simulink model "AirHt_Ctl"  (R2016b)
settings: configuration reference "CodeGenConfigSet" (kept outside this file)
values from neighbouring files (symbols this model uses):
  AirHt_bCEngDsT_C = Calibration.Parameter    [init_AirHt_Ctl.m]    (also in init_AirHt_Ctl_SIL.m = Simulink.Parameter)
  AirHt_bEnvT_C = Calibration.Parameter    [init_AirHt_Ctl.m]    (also in init_AirHt_Ctl_SIL.m = Simulink.Parameter)
  AirHt_bFuelT_C = Calibration.Parameter    [init_AirHt_Ctl.m]    (also in init_AirHt_Ctl_SIL.m = Simulink.Parameter)
  AirHt_bOilT_C = Calibration.Parameter    [init_AirHt_Ctl.m]    (also in init_AirHt_Ctl_SIL.m = Simulink.Parameter)
  AirHt_btAFS_C = Calibration.Parameter    [init_AirHt_Ctl.m]    (also in init_AirHt_Ctl_SIL.m = Simulink.Parameter)
  AirHt_btCACDs_C = Calibration.Parameter    [init_AirHt_Ctl.m]    (also in init_AirHt_Ctl_SIL.m = Simulink.Parameter)
  AirHt_btIntkVUs_C = Calibration.Parameter    [init_AirHt_Ctl.m]    (also in init_AirHt_Ctl_SIL.m = Simulink.Parameter)
  AIRHT_MAX_TEMP = fi(150,Temp_deg)    [init_AirHt_Ctl.m]    (also in init_AirHt_Ctl_SIL.m)
  AirHt_nMin_C = Calibration.Parameter    [init_AirHt_Ctl.m]    (also in init_AirHt_Ctl_SIL.m = Simulink.Parameter)
  AirHt_referencetemp_C = Calibration.Parameter    [init_AirHt_Ctl.m]    (also in init_AirHt_Ctl_SIL.m = Simulink.Parameter)
  AirHt_tiBlink_C = Calibration.Parameter    [init_AirHt_Ctl.m]    (also in init_AirHt_Ctl_SIL.m = Simulink.Parameter)
  AirHt_tiCrankHt_MAP = Calibration.Parameter    [init_AirHt_Ctl.m]    (also in init_AirHt_Ctl_SIL.m = Simulink.Parameter)
  AirHt_tiCrankHt_MAPX = Calibration.Parameter    [init_AirHt_Ctl.m]    (also in init_AirHt_Ctl_SIL.m = Simulink.Parameter)
  AirHt_tiCrankHt_MAPY = Calibration.Parameter    [init_AirHt_Ctl.m]    (also in init_AirHt_Ctl_SIL.m = Simulink.Parameter)
  AirHt_tiLowBattThr_C = Calibration.Parameter    [init_AirHt_Ctl.m]    (also in init_AirHt_Ctl_SIL.m = Simulink.Parameter)
  AirHt_tiPostHt_MAP = Calibration.Parameter    [init_AirHt_Ctl.m]    (also in init_AirHt_Ctl_SIL.m = Simulink.Parameter)
  AirHt_tiPostHt_MAPX = Calibration.Parameter    [init_AirHt_Ctl.m]    (also in init_AirHt_Ctl_SIL.m = Simulink.Parameter)
  AirHt_tiPostHt_MAPY = Calibration.Parameter    [init_AirHt_Ctl.m]    (also in init_AirHt_Ctl_SIL.m = Simulink.Parameter)
  AirHt_tiPreHt_MAP = Calibration.Parameter    [init_AirHt_Ctl.m]    (also in init_AirHt_Ctl_SIL.m = Simulink.Parameter)
  AirHt_tiPreHt_MAPX = Calibration.Parameter    [init_AirHt_Ctl.m]    (also in init_AirHt_Ctl_SIL.m = Simulink.Parameter)
  AirHt_tiPreHt_MAPY = Calibration.Parameter    [init_AirHt_Ctl.m]    (also in init_AirHt_Ctl_SIL.m = Simulink.Parameter)
  AirHt_tiStByHt_MAP = Calibration.Parameter    [init_AirHt_Ctl.m]    (also in init_AirHt_Ctl_SIL.m = Simulink.Parameter)
  AirHt_tiStByHt_MAPX = Calibration.Parameter    [init_AirHt_Ctl.m]    (also in init_AirHt_Ctl_SIL.m = Simulink.Parameter)
  AirHt_tiStByHt_MAPY = Calibration.Parameter    [init_AirHt_Ctl.m]    (also in init_AirHt_Ctl_SIL.m = Simulink.Parameter)
  AirHt_tiStDelay_C = Calibration.Parameter    [init_AirHt_Ctl.m]    (also in init_AirHt_Ctl_SIL.m = Simulink.Parameter)
  AirHt_uLowBattThr_C = Calibration.Parameter    [init_AirHt_Ctl.m]    (also in init_AirHt_Ctl_SIL.m = Simulink.Parameter)
undefined symbols (not defined in the file or in its folder): AirHt_Ctl_DT, AirHtState_conv, EngState_conv
libraries: CXLib x2
settings Model: Creator=GaberXu  LastModifiedBy=guanxiaoxing
settings ConfigSetRef: SourceLocation=Base Workspace

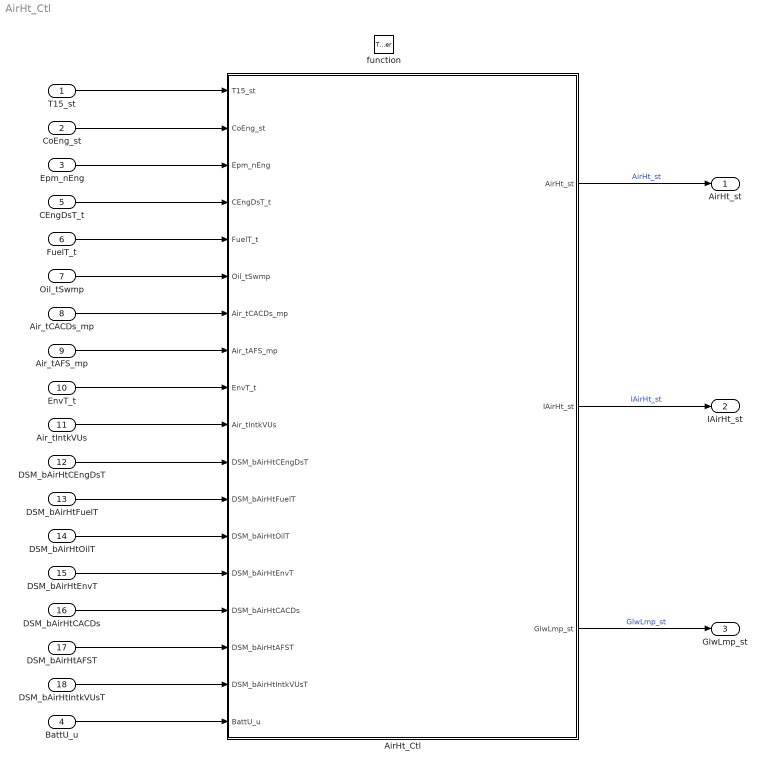
== system AirHt_Ctl ==
  T15_st : Inport  Description=Terminal 15 status after debouncing  OutDataTypeStr=Enum: Switch_conv
  CoEng_st : Inport  Description=Engine coordinator state  Port=2  OutDataTypeStr=Enum: EngState_conv
  Epm_nEng : Inport  Tag=rpm  Description=Engine speed  Port=3  OutMin=0  OutMax=6000  OutDataTypeStr=EngSpeed_rpm
  BattU_u : Inport  Tag=mv  Description=Battery voltage  Port=4  OutMin=0  OutMax=50000  OutDataTypeStr=Battery_mv
  CEngDsT_t : Inport  Tag=deg  Description=engine coolant temperature after filter  Port=5  OutMin=-200  OutMax=200  OutDataTypeStr=Temp_deg
  FuelT_t : Inport  Tag=deg  Description=Temperature of fuel  Port=6  OutMin=-50  OutMax=150  OutDataTypeStr=Temp_deg
  Oil_tSwmp : Inport  Tag=deg  Description=Oil temperature in oil sump  Port=7  OutMin=-50  OutMax=200  OutDataTypeStr=Temp_deg
  Air_tCACDs_mp : Inport  Tag=deg  Description=Charge-air temperature downstream from charge-air cooler  Port=8  OutMin=-200  OutMax=200  OutDataTypeStr=Temp_deg
  Air_tAFS_mp : Inport  Tag=deg  Description=Induction air temperature at the HFM  Port=9  OutMin=-200  OutMax=200  OutDataTypeStr=Temp_deg
  EnvT_t : Inport  Tag=deg  Description=Environmental temperature  Port=10  OutMin=-200  OutMax=200  OutDataTypeStr=Temp_deg
  Air_tIntkVUs : Inport  Tag=deg  Description=Intake air temperature upstream of the inlet valve  Port=11  OutMin=-200  OutMax=200  OutDataTypeStr=Temp_deg
  DSM_bAirHtCEngDsT : Inport  Description=Status of FId_AirHtCEngDsT  Port=12  OutMin=0  OutMax=1  OutDataTypeStr=boolean
  DSM_bAirHtFuelT : Inport  Description=Status of FId_AirHtFuelT  Port=13  OutMin=0  OutMax=1  OutDataTypeStr=boolean
  DSM_bAirHtOilT : Inport  Description=Status of FId_AirHtOilT  Port=14  OutMin=0  OutMax=1  OutDataTypeStr=boolean
  DSM_bAirHtEnvT : Inport  Description=Status of FId_AirHtEnvT_mp  Port=15  OutMin=0  OutMax=1  OutDataTypeStr=boolean
  DSM_bAirHtCACDs : Inport  Description=Status of FId_AirHtCACDs  Port=16  OutMin=0  OutMax=1  OutDataTypeStr=boolean
  DSM_bAirHtAFST : Inport  Description=Status of FId_AirHtAFST  Port=17  OutMin=0  OutMax=1  OutDataTypeStr=boolean
  DSM_bAirHtIntkVUsT : Inport  Description=Status of FId_AirHtntkVUsT  Port=18  OutMin=0  OutMax=1  OutDataTypeStr=boolean
  function : TriggerPort  TriggerType=function-call  VariantControl=Variant  PortDimensions=1
  AirHt_Ctl : Subsystem
  AirHt_st : Outport  Description=status of AirHeater  OutDataTypeStr=Enum: AirHtState_conv
  IAirHt_st : Outport  Description=Request for intake air heater ON/OFF from ASW.  Port=2  OutMin=0  OutMax=1  OutDataTypeStr=boolean
  GlwLmp_st : Outport  Description=Glow lamp status  Port=3  OutMin=0  OutMax=1  OutDataTypeStr=boolean
  wires:
  AirHt_Ctl/1(AirHt_st) -> AirHt_st/1  "AirHt_st"
  AirHt_Ctl/2(IAirHt_st) -> IAirHt_st/1  "IAirHt_st"
  AirHt_Ctl/3(GlwLmp_st) -> GlwLmp_st/1  "GlwLmp_st"
  CoEng_st/1 -> AirHt_Ctl/2(CoEng_st)
  Epm_nEng/1 -> AirHt_Ctl/3(Epm_nEng)
  T15_st/1 -> AirHt_Ctl/1(T15_st)
  BattU_u/1 -> AirHt_Ctl/18(BattU_u)
  CEngDsT_t/1 -> AirHt_Ctl/4(CEngDsT_t)
  DSM_bAirHtIntkVUsT/1 -> AirHt_Ctl/17(DSM_bAirHtIntkVUsT)
  DSM_bAirHtEnvT/1 -> AirHt_Ctl/14(DSM_bAirHtEnvT)
  DSM_bAirHtCACDs/1 -> AirHt_Ctl/15(DSM_bAirHtCACDs)
  Oil_tSwmp/1 -> AirHt_Ctl/6(Oil_tSwmp)
  Air_tAFS_mp/1 -> AirHt_Ctl/8(Air_tAFS_mp)
  DSM_bAirHtAFST/1 -> AirHt_Ctl/16(DSM_bAirHtAFST)
  DSM_bAirHtFuelT/1 -> AirHt_Ctl/12(DSM_bAirHtFuelT)
  FuelT_t/1 -> AirHt_Ctl/5(FuelT_t)
  Air_tIntkVUs/1 -> AirHt_Ctl/10(Air_tIntkVUs)
  Air_tCACDs_mp/1 -> AirHt_Ctl/7(Air_tCACDs_mp)
  EnvT_t/1 -> AirHt_Ctl/9(EnvT_t)
  DSM_bAirHtOilT/1 -> AirHt_Ctl/13(DSM_bAirHtOilT)
  DSM_bAirHtCEngDsT/1 -> AirHt_Ctl/11(DSM_bAirHtCEngDsT)

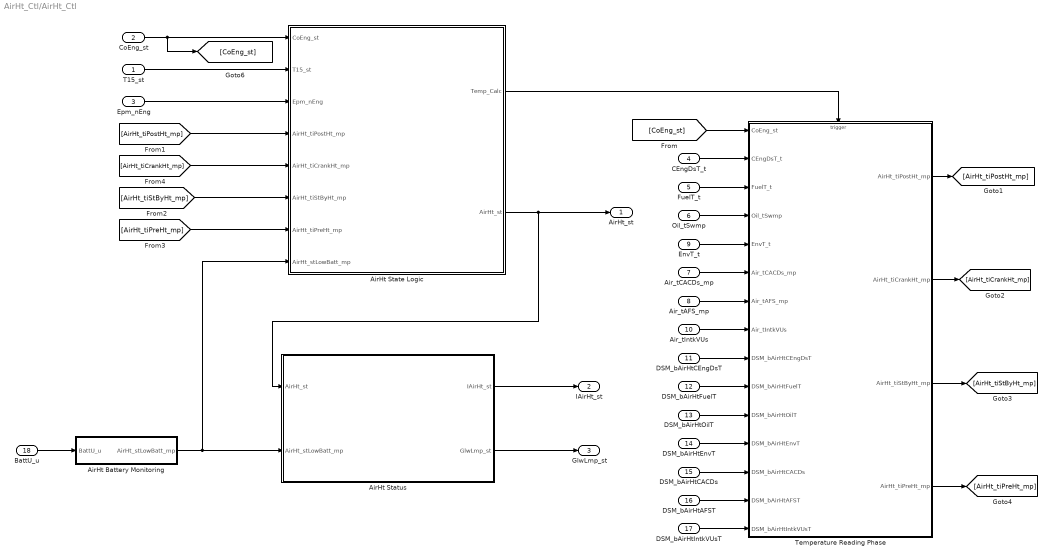
== system AirHt_Ctl/AirHt_Ctl ==
  T15_st : Inport  Description=Terminal 15 status after debouncing
  CoEng_st : Inport  Description=Engine coordinator state  Port=2
  Epm_nEng : Inport  Tag=rpm  Description=Engine speed  Port=3
  CEngDsT_t : Inport  Tag=deg  Description=engine coolant temperature after filter  Port=4  OutMin=-200  OutMax=200  OutDataTypeStr=Temp_deg
  FuelT_t : Inport  Tag=deg  Description=Temperature of fuel  Port=5  OutMin=-50  OutMax=150  OutDataTypeStr=Temp_deg
  Oil_tSwmp : Inport  Tag=deg  Description=Oil temperature in oil sump  Port=6  OutMin=-50  OutMax=200  OutDataTypeStr=Temp_deg
  Air_tCACDs_mp : Inport  Tag=deg  Description=Charge-air temperature downstream from charge-air cooler  Port=7  OutMin=-200  OutMax=200  OutDataTypeStr=Temp_deg
  Air_tAFS_mp : Inport  Tag=deg  Description=Induction air temperature at the HFM  Port=8  OutMin=-200  OutMax=200  OutDataTypeStr=Temp_deg
  EnvT_t : Inport  Tag=deg  Description=Environmental temperature  Port=9  OutMin=-200  OutMax=200  OutDataTypeStr=Temp_deg
  Air_tIntkVUs : Inport  Tag=deg  Description=Intake air temperature upstream of the inlet valve  Port=10  OutMin=-200  OutMax=200  OutDataTypeStr=Temp_deg
  DSM_bAirHtCEngDsT : Inport  Description=Status of FId_AirHtCEngDsT  Port=11  OutMin=0  OutMax=1  OutDataTypeStr=boolean
  DSM_bAirHtFuelT : Inport  Description=Status of FId_AirHtFuelT  Port=12  OutMin=0  OutMax=1  OutDataTypeStr=boolean
  DSM_bAirHtOilT : Inport  Description=Status of FId_AirHtOilT  Port=13  OutMin=0  OutMax=1  OutDataTypeStr=boolean
  DSM_bAirHtEnvT : Inport  Description=Status of FId_AirHtEnvT_mp  Port=14  OutMin=0  OutMax=1  OutDataTypeStr=boolean
  DSM_bAirHtCACDs : Inport  Description=Status of FId_AirHtCACDs  Port=15  OutMin=0  OutMax=1  OutDataTypeStr=boolean
  DSM_bAirHtAFST : Inport  Description=Status of FId_AirHtAFST  Port=16  OutMin=0  OutMax=1  OutDataTypeStr=boolean
  DSM_bAirHtIntkVUsT : Inport  Description=Status of FId_AirHtntkVUsT  Port=17  OutMin=0  OutMax=1  OutDataTypeStr=boolean
  BattU_u : Inport  Tag=mv  Description=Battery voltage  Port=18
  AirHt Battery Monitoring : Subsystem
  AirHt State Logic : Subsystem
  AirHt Status : Subsystem
  Temperature Reading Phase : Subsystem
      settings: RTWFcnNameOpts=User specified  RTWFileNameOpts=User specified
  AirHt_st : Outport  Description=status of AirHeater
  IAirHt_st : Outport  Description=Request for intake air heater ON/OFF from ASW.  Port=2
  GlwLmp_st : Outport  Description=Glow lamp status  Port=3
  wires:
  T15_st/1 -> AirHt State Logic/2(T15_st)
  Epm_nEng/1 -> AirHt State Logic/3(Epm_nEng)
  [AirHt_tiStByHt_mp] -> AirHt State Logic/6(AirHt_tiStByHt_mp)
  [AirHt_tiPostHt_mp] -> AirHt State Logic/4(AirHt_tiPostHt_mp)
  [AirHt_tiCrankHt_mp] -> AirHt State Logic/5(AirHt_tiCrankHt_mp)
  AirHt Status/1(IAirHt_st) -> IAirHt_st/1
  AirHt Status/2(GlwLmp_st) -> GlwLmp_st/1
  CoEng_st/1 -> [CoEng_st], AirHt State Logic/1(CoEng_st)
  Temperature Reading Phase/1(AirHt_tiPostHt_mp) -> [AirHt_tiPostHt_mp]
  Temperature Reading Phase/2(AirHt_tiCrankHt_mp) -> [AirHt_tiCrankHt_mp]
  Temperature Reading Phase/3(AirHt_tiStByHt_mp) -> [AirHt_tiStByHt_mp]
  Temperature Reading Phase/4(AirHt_tiPreHt_mp) -> [AirHt_tiPreHt_mp]
  AirHt State Logic/2(AirHt_st) -> AirHt_st/1, AirHt Status/1(AirHt_st)
  AirHt State Logic/1(Temp_Calc) -> Temperature Reading Phase/Trigger
  [CoEng_st] -> Temperature Reading Phase/1(CoEng_st)
  CEngDsT_t/1 -> Temperature Reading Phase/2(CEngDsT_t)
  DSM_bAirHtOilT/1 -> Temperature Reading Phase/11(DSM_bAirHtOilT)
  DSM_bAirHtCACDs/1 -> Temperature Reading Phase/13(DSM_bAirHtCACDs)
  Oil_tSwmp/1 -> Temperature Reading Phase/4(Oil_tSwmp)
  DSM_bAirHtCEngDsT/1 -> Temperature Reading Phase/9(DSM_bAirHtCEngDsT)
  DSM_bAirHtEnvT/1 -> Temperature Reading Phase/12(DSM_bAirHtEnvT)
  DSM_bAirHtAFST/1 -> Temperature Reading Phase/14(DSM_bAirHtAFST)
  DSM_bAirHtIntkVUsT/1 -> Temperature Reading Phase/15(DSM_bAirHtIntkVUsT)
  DSM_bAirHtFuelT/1 -> Temperature Reading Phase/10(DSM_bAirHtFuelT)
  Air_tIntkVUs/1 -> Temperature Reading Phase/8(Air_tIntkVUs)
  FuelT_t/1 -> Temperature Reading Phase/3(FuelT_t)
  AirHt Battery Monitoring/1(AirHt_stLowBatt_mp) -> AirHt State Logic/8(AirHt_stLowBatt_mp), AirHt Status/2(AirHt_stLowBatt_mp)
  BattU_u/1 -> AirHt Battery Monitoring/1(BattU_u)
  [AirHt_tiPreHt_mp] -> AirHt State Logic/7(AirHt_tiPreHt_mp)
  EnvT_t/1 -> Temperature Reading Phase/5(EnvT_t)
  Air_tAFS_mp/1 -> Temperature Reading Phase/7(Air_tAFS_mp)
  Air_tCACDs_mp/1 -> Temperature Reading Phase/6(Air_tCACDs_mp)

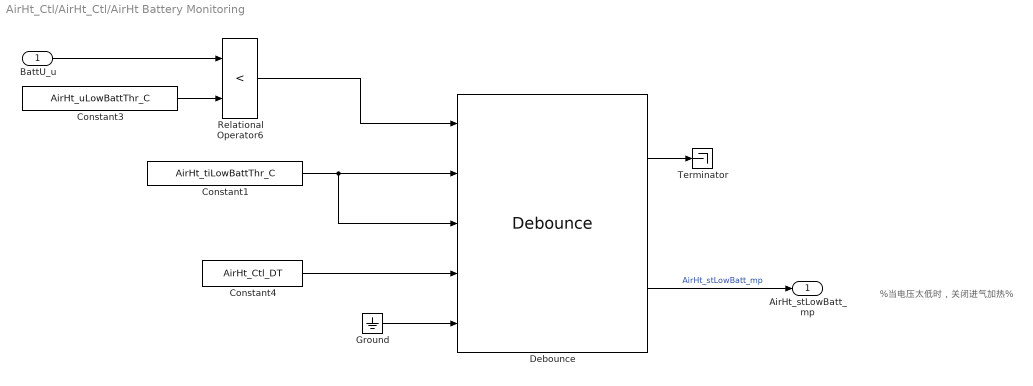
== system AirHt_Ctl/AirHt_Ctl/AirHt Battery Monitoring ==
  note: %当电压太低时，关闭进气加热%
  BattU_u : Inport
  Constant1 : Constant  Value=AirHt_tiLowBattThr_C  SampleTime=-1
  Constant3 : Constant  Value=AirHt_uLowBattThr_C  SampleTime=-1
  Constant4 : Constant  Value=AirHt_Ctl_DT  SampleTime=-1
  Debounce : CXLib/Debounce
  Ground : Ground
  Relational Operator6 : RelationalOperator  Operator=<  OutDataTypeStr=boolean  RndMeth=Simplest  InputSameDT=on
  Terminator : Terminator
  AirHt_stLowBatt_mp : Outport
  wires:
  Relational Operator6/1 -> Debounce/1
  BattU_u/1 -> Relational Operator6/1
  Debounce/1 -> Terminator/1
  Debounce/2 -> AirHt_stLowBatt_mp/1  "AirHt_stLowBatt_mp"
  Constant1/1 -> Debounce/2, Debounce/3
  Ground/1 -> Debounce/5
  Constant3/1 -> Relational Operator6/2
  Constant4/1 -> Debounce/4

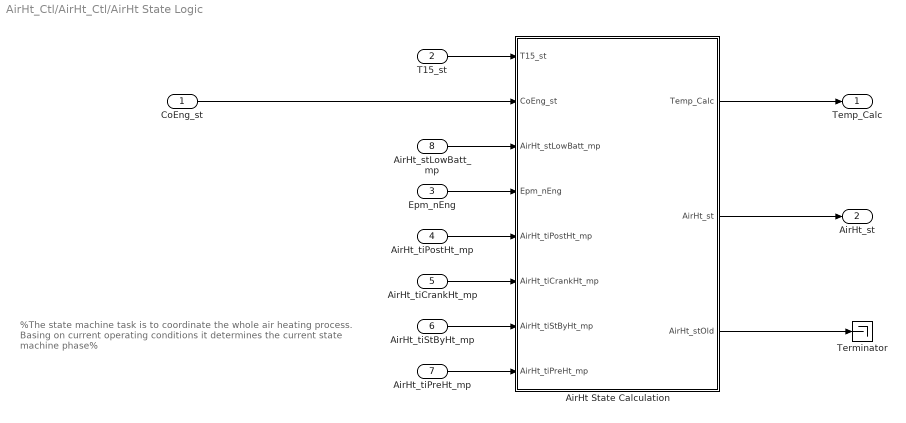
== system AirHt_Ctl/AirHt_Ctl/AirHt State Logic ==
  note: %The state machine task is to coordinate the whole air heating process.
      | Basing on current operating conditions it determines the current state
      | machine phase%
  CoEng_st : Inport
  T15_st : Inport  Port=2
  Epm_nEng : Inport  Port=3
  AirHt_tiPostHt_mp : Inport  Port=4
  AirHt_tiCrankHt_mp : Inport  Port=5
  AirHt_tiStByHt_mp : Inport  Port=6
  AirHt_tiPreHt_mp : Inport  Port=7
  AirHt_stLowBatt_mp : Inport  Port=8
  AirHt State Calculation : Subsystem
      settings: RTWFcnNameOpts=User specified  RTWFileNameOpts=User specified
  Terminator : Terminator
  Temp_Calc : Outport
  AirHt_st : Outport  Port=2
  wires:
  AirHt State Calculation/3(AirHt_stOld) -> Terminator/1
  Epm_nEng/1 -> AirHt State Calculation/4(Epm_nEng)
  AirHt_stLowBatt_mp/1 -> AirHt State Calculation/3(AirHt_stLowBatt_mp)
  T15_st/1 -> AirHt State Calculation/1(T15_st)
  AirHt State Calculation/2(AirHt_st) -> AirHt_st/1
  AirHt_tiPostHt_mp/1 -> AirHt State Calculation/5(AirHt_tiPostHt_mp)
  AirHt_tiCrankHt_mp/1 -> AirHt State Calculation/6(AirHt_tiCrankHt_mp)
  AirHt_tiStByHt_mp/1 -> AirHt State Calculation/7(AirHt_tiStByHt_mp)
  AirHt_tiPreHt_mp/1 -> AirHt State Calculation/8(AirHt_tiPreHt_mp)
  CoEng_st/1 -> AirHt State Calculation/2(CoEng_st)
  AirHt State Calculation/1(Temp_Calc) -> Temp_Calc/1

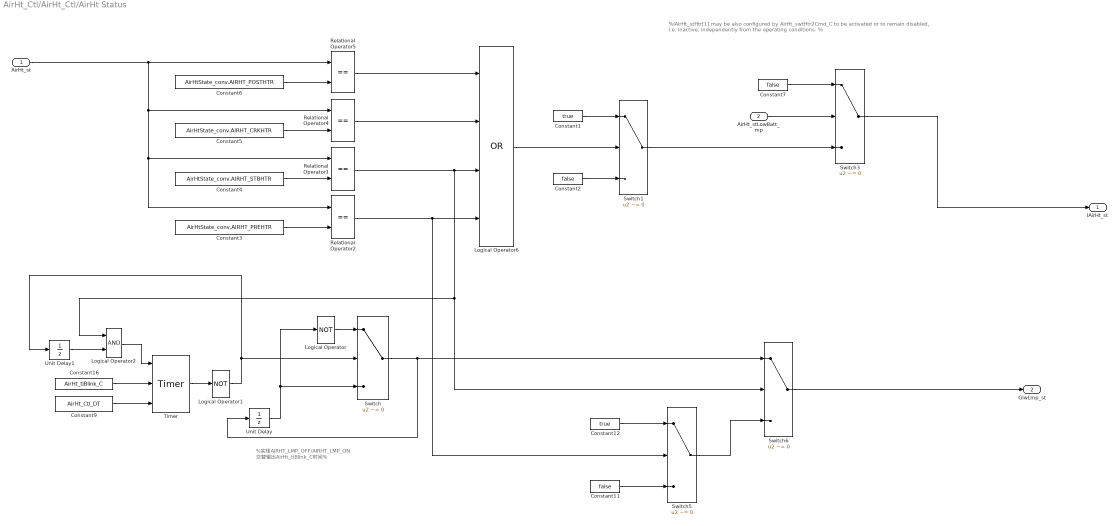
== system AirHt_Ctl/AirHt_Ctl/AirHt Status ==
  note: %实现AIRHT_LMP_OFF/AIRHT_LMP_ON
      | 交替输出AirHt_tiBlink_C时间%
  note: %IAirHt_stHtr[1] may be also configured by AirHt_swtHtr2Cmd_C to be activated or to remain disabled, i.e. inactive, independently
      | from the operating conditions. %
  AirHt_st : Inport
  AirHt_stLowBatt_mp : Inport  Port=2
  Constant1 : Constant  Value=true  OutDataTypeStr=boolean
  Constant11 : Constant  Value=false  OutDataTypeStr=boolean
  Constant12 : Constant  Value=true  OutDataTypeStr=boolean
  Constant16 : Constant  Value=AirHt_tiBlink_C  SampleTime=-1
  Constant2 : Constant  Value=false  OutDataTypeStr=boolean
  Constant3 : Constant  Value=AirHtState_conv.AIRHT_PREHTR  SampleTime=-1
  Constant4 : Constant  Value=AirHtState_conv.AIRHT_STBHTR  SampleTime=-1
  Constant5 : Constant  Value=AirHtState_conv.AIRHT_CRKHTR  SampleTime=-1
  Constant6 : Constant  Value=AirHtState_conv.AIRHT_POSTHTR  SampleTime=-1
  Constant7 : Constant  Value=false  OutDataTypeStr=boolean
  Constant9 : Constant  Value=AirHt_Ctl_DT  SampleTime=-1
  Logical Operator : Logic  Operator=NOT  AllPortsSameDT=off  OutDataTypeStr=boolean
  Logical Operator1 : Logic  Operator=NOT  AllPortsSameDT=off  OutDataTypeStr=boolean
  Logical Operator2 : Logic  AllPortsSameDT=off  OutDataTypeStr=boolean
  Logical Operator6 : Logic  Operator=OR  Inputs=4  OutDataTypeStr=boolean
  Relational Operator{1..2,4..5} (4 alike) : RelationalOperator  Operator===  OutDataTypeStr=boolean  RndMeth=Simplest  InputSameDT=on
  Switch : Switch  Criteria=u2 ~= 0
  Switch1 : Switch  Criteria=u2 ~= 0  InputSameDT=on
  Switch3 : Switch  Criteria=u2 ~= 0  SaturateOnIntegerOverflow=on  InputSameDT=on
  Switch5 : Switch  Criteria=u2 ~= 0  SaturateOnIntegerOverflow=on  InputSameDT=on
  Switch6 : Switch  Criteria=u2 ~= 0  SaturateOnIntegerOverflow=on  InputSameDT=on
  Timer : CXLib/Timer
  Unit Delay : UnitDelay  SampleTime=-1
      settings: AttributesFormatString=InitialValue=%<InitialCondition>
  Unit Delay1 : UnitDelay  SampleTime=-1
      settings: AttributesFormatString=InitialValue=%<InitialCondition>
  IAirHt_st : Outport  Description=Request for intake air heater ON/OFF from ASW.
  GlwLmp_st : Outport  Description=Glow lamp status  Port=2
  wires:
  Switch6/1 -> GlwLmp_st/1
  Switch3/1 -> IAirHt_st/1
  Logical Operator/1 -> Switch/1
  Unit Delay1/1 -> Logical Operator2/2
  Logical Operator1/1 -> Switch/2, Unit Delay1/1
  Switch/1 -> Unit Delay/1, Switch6/1
  Timer/1 -> Logical Operator1/1
  Unit Delay/1 -> Switch/3, Logical Operator/1
  Constant16/1 -> Timer/2
  Constant9/1 -> Timer/3
  AirHt_st/1 -> Relational Operator1/1, Relational Operator2/1, Relational Operator4/1, Relational Operator5/1
  Constant4/1 -> Relational Operator1/2
  Constant3/1 -> Relational Operator2/2
  Constant5/1 -> Relational Operator4/2
  Constant6/1 -> Relational Operator5/2
  Relational Operator5/1 -> Logical Operator6/1
  Logical Operator6/1 -> Switch1/2
  AirHt_stLowBatt_mp/1 -> Switch3/2
  Switch1/1 -> Switch3/3
  Relational Operator2/1 -> Logical Operator6/4, Switch5/2
  Constant11/1 -> Switch5/3
  Constant12/1 -> Switch5/1
  Relational Operator4/1 -> Logical Operator6/2
  Switch5/1 -> Switch6/3
  Constant7/1 -> Switch3/1
  Constant1/1 -> Switch1/1
  Constant2/1 -> Switch1/3
  Relational Operator1/1 -> Logical Operator6/3, Logical Operator2/1, Switch6/2
  Logical Operator2/1 -> Timer/1

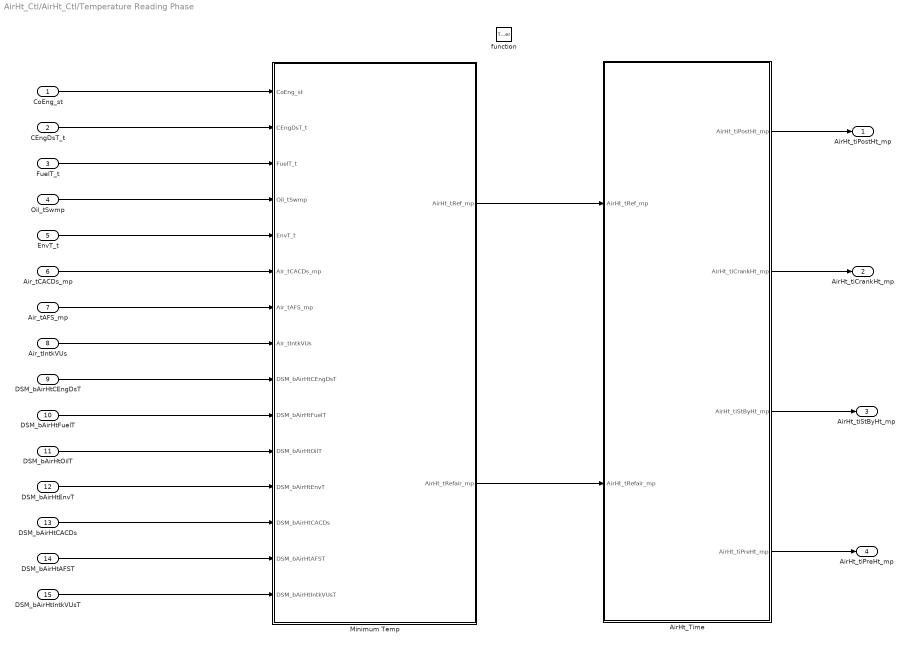
== system AirHt_Ctl/AirHt_Ctl/Temperature Reading Phase ==
  CoEng_st : Inport
  CEngDsT_t : Inport  Port=2
  FuelT_t : Inport  Port=3
  Oil_tSwmp : Inport  Port=4
  EnvT_t : Inport  Port=5
  Air_tCACDs_mp : Inport  Tag=deg  Description=Charge-air temperature downstream from charge-air cooler  Port=6
  Air_tAFS_mp : Inport  Tag=deg  Description=Induction air temperature at the HFM  Port=7
  Air_tIntkVUs : Inport  Tag=deg  Description=Intake air temperature upstream of the inlet valve  Port=8
  DSM_bAirHtCEngDsT : Inport  Description=Status of FId_AirHtCEngDsT  Port=9
  DSM_bAirHtFuelT : Inport  Description=Status of FId_AirHtFuelT  Port=10
  DSM_bAirHtOilT : Inport  Description=Status of FId_AirHtOilT  Port=11
  DSM_bAirHtEnvT : Inport  Description=Status of FId_AirHtEnvT_mp  Port=12
  DSM_bAirHtCACDs : Inport  Description=Status of FId_AirHtCACDs  Port=13
  DSM_bAirHtAFST : Inport  Description=Status of FId_AirHtEnvT_mp  Port=14
  DSM_bAirHtIntkVUsT : Inport  Description=Status of FId_AirHtCACDs  Port=15
  function : TriggerPort  TriggerType=function-call  VariantControl=Variant
  AirHt_Time : Subsystem
  Minimum Temp : Subsystem
  AirHt_tiPostHt_mp : Outport
  AirHt_tiCrankHt_mp : Outport  Port=2
  AirHt_tiStByHt_mp : Outport  Port=3
  AirHt_tiPreHt_mp : Outport  Port=4
  wires:
  CoEng_st/1 -> Minimum Temp/1(CoEng_st)
  CEngDsT_t/1 -> Minimum Temp/2(CEngDsT_t)
  FuelT_t/1 -> Minimum Temp/3(FuelT_t)
  Oil_tSwmp/1 -> Minimum Temp/4(Oil_tSwmp)
  EnvT_t/1 -> Minimum Temp/5(EnvT_t)
  Air_tCACDs_mp/1 -> Minimum Temp/6(Air_tCACDs_mp)
  Air_tAFS_mp/1 -> Minimum Temp/7(Air_tAFS_mp)
  Air_tIntkVUs/1 -> Minimum Temp/8(Air_tIntkVUs)
  DSM_bAirHtCEngDsT/1 -> Minimum Temp/9(DSM_bAirHtCEngDsT)
  DSM_bAirHtFuelT/1 -> Minimum Temp/10(DSM_bAirHtFuelT)
  DSM_bAirHtOilT/1 -> Minimum Temp/11(DSM_bAirHtOilT)
  DSM_bAirHtEnvT/1 -> Minimum Temp/12(DSM_bAirHtEnvT)
  DSM_bAirHtCACDs/1 -> Minimum Temp/13(DSM_bAirHtCACDs)
  DSM_bAirHtAFST/1 -> Minimum Temp/14(DSM_bAirHtAFST)
  DSM_bAirHtIntkVUsT/1 -> Minimum Temp/15(DSM_bAirHtIntkVUsT)
  Minimum Temp/1(AirHt_tRef_mp) -> AirHt_Time/1(AirHt_tRef_mp)
  Minimum Temp/2(AirHt_tRefair_mp) -> AirHt_Time/2(AirHt_tRefair_mp)
  AirHt_Time/3(AirHt_tiStByHt_mp) -> AirHt_tiStByHt_mp/1
  AirHt_Time/1(AirHt_tiPostHt_mp) -> AirHt_tiPostHt_mp/1
  AirHt_Time/2(AirHt_tiCrankHt_mp) -> AirHt_tiCrankHt_mp/1
  AirHt_Time/4(AirHt_tiPreHt_mp) -> AirHt_tiPreHt_mp/1

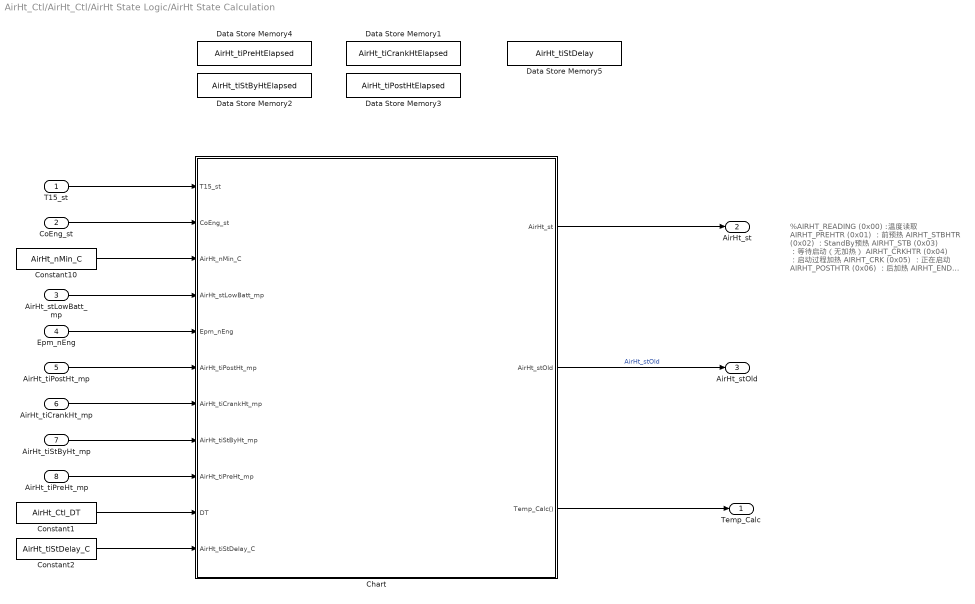
== system AirHt_Ctl/AirHt_Ctl/AirHt State Logic/AirHt State Calculation ==
  note: %AIRHT_READING (0x00) :温度读取
      | AIRHT_PREHTR (0x01) ：前预热
      | AIRHT_STBHTR (0x02) ：StandBy预热
      | AIRHT_STB (0x03) ：等待启动（无加热）
      | AIRHT_CRKHTR (0x04) ：启动过程加热
      | AIRHT_CRK (0x05) ：正在启动
      | AIRHT_POSTHTR (0x06) ：后加热
      | AIRHT_END (0x07) ：加热完成
      | AIRHT_AFTERRUN (0x08) ：afterrun模式%
  T15_st : Inport
  CoEng_st : Inport  Port=2
  AirHt_stLowBatt_mp : Inport  Port=3
  Epm_nEng : Inport  Port=4
  AirHt_tiPostHt_mp : Inport  Port=5
  AirHt_tiCrankHt_mp : Inport  Port=6
  AirHt_tiStByHt_mp : Inport  Port=7
  AirHt_tiPreHt_mp : Inport  Port=8
  Chart : Stateflow chart  TreatAsAtomicUnit=on
  Constant1 : Constant  Value=AirHt_Ctl_DT  SampleTime=-1
  Constant10 : Constant  Value=AirHt_nMin_C  SampleTime=-1
  Constant2 : Constant  Value=AirHt_tiStDelay_C  SampleTime=-1
  Data Store Memory1 : DataStoreMemory  DataStoreName=AirHt_tiCrankHtElapsed  ReadBeforeWriteMsg=warning  WriteAfterWriteMsg=warning  WriteAfterReadMsg=warning  ShowAdditionalParam=off  StateMustResolveToSignalObject=on
  Data Store Memory2 : DataStoreMemory  DataStoreName=AirHt_tiStByHtElapsed  ReadBeforeWriteMsg=warning  WriteAfterWriteMsg=warning  WriteAfterReadMsg=warning  ShowAdditionalParam=off  StateMustResolveToSignalObject=on
  Data Store Memory3 : DataStoreMemory  DataStoreName=AirHt_tiPostHtElapsed  ReadBeforeWriteMsg=warning  WriteAfterWriteMsg=warning  WriteAfterReadMsg=warning  ShowAdditionalParam=off  StateMustResolveToSignalObject=on
  Data Store Memory4 : DataStoreMemory  DataStoreName=AirHt_tiPreHtElapsed  ReadBeforeWriteMsg=warning  WriteAfterWriteMsg=warning  WriteAfterReadMsg=warning  ShowAdditionalParam=off  StateMustResolveToSignalObject=on
  Data Store Memory5 : DataStoreMemory  DataStoreName=AirHt_tiStDelay  ReadBeforeWriteMsg=warning  WriteAfterWriteMsg=warning  WriteAfterReadMsg=warning  ShowAdditionalParam=off  StateMustResolveToSignalObject=on
  Temp_Calc : Outport
  AirHt_st : Outport  Port=2
  AirHt_stOld : Outport  Port=3
  wires:
  CoEng_st/1 -> Chart/2(CoEng_st)
  AirHt_tiStByHt_mp/1 -> Chart/8(AirHt_tiStByHt_mp)
  AirHt_tiCrankHt_mp/1 -> Chart/7(AirHt_tiCrankHt_mp)
  Constant10/1 -> Chart/3(AirHt_nMin_C)
  Epm_nEng/1 -> Chart/5(Epm_nEng)
  Constant1/1 -> Chart/10(DT)
  T15_st/1 -> Chart/1(T15_st)
  Chart/2(AirHt_stOld) -> AirHt_stOld/1  "AirHt_stOld"
  Chart/1(AirHt_st) -> AirHt_st/1
  AirHt_tiPostHt_mp/1 -> Chart/6(AirHt_tiPostHt_mp)
  AirHt_stLowBatt_mp/1 -> Chart/4(AirHt_stLowBatt_mp)
  AirHt_tiPreHt_mp/1 -> Chart/9(AirHt_tiPreHt_mp)
  Chart/3(Temp_Calc()) -> Temp_Calc/1
  Constant2/1 -> Chart/11(AirHt_tiStDelay_C)

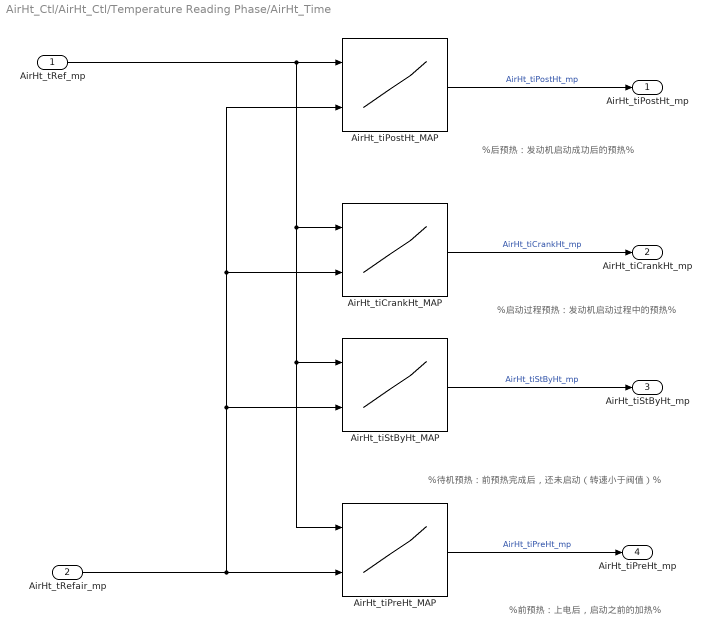
== system AirHt_Ctl/AirHt_Ctl/Temperature Reading Phase/AirHt_Time ==
  note: %前预热：上电后，启动之前的加热%
  note: %待机预热：前预热完成后，还未启动（转速小于阀值）%
  note: %启动过程预热：发动机启动过程中的预热%
  note: %后预热：发动机启动成功后的预热%
  AirHt_tRef_mp : Inport  Description=Status of FId_AirHtEnvT_mp
  AirHt_tRefair_mp : Inport  Description=Status of FId_AirHtEnvT_mp  Port=2
  AirHt_tiCrankHt_MAP : Lookup_n-D  DialogController=Simulink.DDGSource  BreakpointsForDimension1=AirHt_tiCrankHt_MAPY  BreakpointsForDimension2=AirHt_tiCrankHt_MAPX  IndexSearchMethod=Linear search  BeginIndexSearchUsingPreviousIndexResult=on  Table=AirHt_tiCrankHt_MAP  ExtrapMethod=Clip  UseLastTableValue=on  InternalRulePriority=Speed  OutDataTypeStr=Inherit: Inherit via back propagation  SaturateOnIntegerOverflow=on
  AirHt_tiPostHt_MAP : Lookup_n-D  DialogController=Simulink.DDGSource  BreakpointsForDimension1=AirHt_tiPostHt_MAPY  BreakpointsForDimension2=AirHt_tiPostHt_MAPX  IndexSearchMethod=Linear search  BeginIndexSearchUsingPreviousIndexResult=on  Table=AirHt_tiPostHt_MAP  ExtrapMethod=Clip  UseLastTableValue=on  InternalRulePriority=Speed  OutDataTypeStr=Inherit: Inherit via back propagation  SaturateOnIntegerOverflow=on
  AirHt_tiPreHt_MAP : Lookup_n-D  DialogController=Simulink.DDGSource  BreakpointsForDimension1=AirHt_tiPreHt_MAPY  BreakpointsForDimension2=AirHt_tiPreHt_MAPX  IndexSearchMethod=Linear search  BeginIndexSearchUsingPreviousIndexResult=on  Table=AirHt_tiPreHt_MAP  ExtrapMethod=Clip  UseLastTableValue=on  InternalRulePriority=Speed  OutDataTypeStr=Inherit: Inherit via back propagation  SaturateOnIntegerOverflow=on
  AirHt_tiStByHt_MAP : Lookup_n-D  DialogController=Simulink.DDGSource  BreakpointsForDimension1=AirHt_tiStByHt_MAPY  BreakpointsForDimension2=AirHt_tiStByHt_MAPX  IndexSearchMethod=Linear search  BeginIndexSearchUsingPreviousIndexResult=on  Table=AirHt_tiStByHt_MAP  ExtrapMethod=Clip  UseLastTableValue=on  InternalRulePriority=Speed  OutDataTypeStr=Inherit: Inherit via back propagation  SaturateOnIntegerOverflow=on
  AirHt_tiPostHt_mp : Outport
  AirHt_tiCrankHt_mp : Outport  Port=2
  AirHt_tiStByHt_mp : Outport  Port=3
  AirHt_tiPreHt_mp : Outport  Port=4
  wires:
  AirHt_tRef_mp/1 -> AirHt_tiPreHt_MAP/1, AirHt_tiStByHt_MAP/1, AirHt_tiCrankHt_MAP/1, AirHt_tiPostHt_MAP/1
  AirHt_tiPreHt_MAP/1 -> AirHt_tiPreHt_mp/1  "AirHt_tiPreHt_mp"
  AirHt_tiCrankHt_MAP/1 -> AirHt_tiCrankHt_mp/1  "AirHt_tiCrankHt_mp"
  AirHt_tRefair_mp/1 -> AirHt_tiStByHt_MAP/2, AirHt_tiPostHt_MAP/2, AirHt_tiCrankHt_MAP/2, AirHt_tiPreHt_MAP/2
  AirHt_tiStByHt_MAP/1 -> AirHt_tiStByHt_mp/1  "AirHt_tiStByHt_mp"
  AirHt_tiPostHt_MAP/1 -> AirHt_tiPostHt_mp/1  "AirHt_tiPostHt_mp"

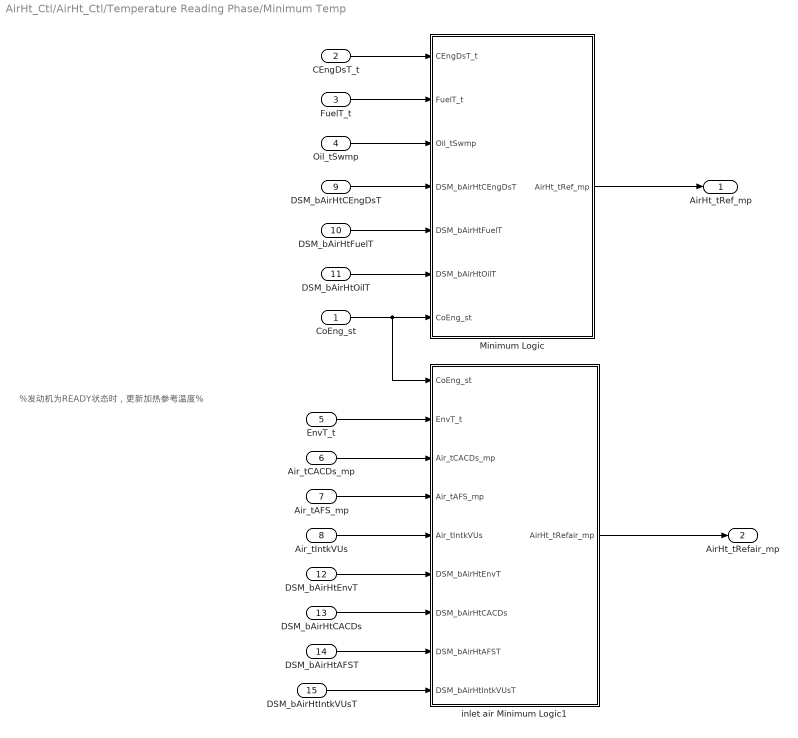
== system AirHt_Ctl/AirHt_Ctl/Temperature Reading Phase/Minimum Temp ==
  note: %发动机为READY状态时，更新加热参考温度%
  CoEng_st : Inport
  CEngDsT_t : Inport  Port=2
  FuelT_t : Inport  Port=3
  Oil_tSwmp : Inport  Port=4
  EnvT_t : Inport  Port=5
  Air_tCACDs_mp : Inport  Tag=deg  Description=Charge-air temperature downstream from charge-air cooler  Port=6
  Air_tAFS_mp : Inport  Tag=deg  Description=Induction air temperature at the HFM  Port=7
  Air_tIntkVUs : Inport  Tag=deg  Description=Intake air temperature upstream of the inlet valve  Port=8
  DSM_bAirHtCEngDsT : Inport  Description=Status of FId_AirHtCEngDsT  Port=9
  DSM_bAirHtFuelT : Inport  Description=Status of FId_AirHtFuelT  Port=10
  DSM_bAirHtOilT : Inport  Description=Status of FId_AirHtOilT  Port=11
  DSM_bAirHtEnvT : Inport  Description=Status of FId_AirHtEnvT_mp  Port=12
  DSM_bAirHtCACDs : Inport  Description=Status of FId_AirHtCACDs  Port=13
  DSM_bAirHtAFST : Inport  Description=Status of FId_AirHtEnvT_mp  Port=14
  DSM_bAirHtIntkVUsT : Inport  Description=Status of FId_AirHtCACDs  Port=15
  Minimum Logic : Subsystem
  inlet air Minimum Logic1 : Subsystem
  AirHt_tRef_mp : Outport
  AirHt_tRefair_mp : Outport  Port=2
  wires:
  DSM_bAirHtOilT/1 -> Minimum Logic/6(DSM_bAirHtOilT)
  CoEng_st/1 -> inlet air Minimum Logic1/1(CoEng_st), Minimum Logic/7(CoEng_st)
  DSM_bAirHtFuelT/1 -> Minimum Logic/5(DSM_bAirHtFuelT)
  DSM_bAirHtIntkVUsT/1 -> inlet air Minimum Logic1/9(DSM_bAirHtIntkVUsT)
  DSM_bAirHtEnvT/1 -> inlet air Minimum Logic1/6(DSM_bAirHtEnvT)
  DSM_bAirHtCACDs/1 -> inlet air Minimum Logic1/7(DSM_bAirHtCACDs)
  EnvT_t/1 -> inlet air Minimum Logic1/2(EnvT_t)
  Oil_tSwmp/1 -> Minimum Logic/3(Oil_tSwmp)
  Air_tAFS_mp/1 -> inlet air Minimum Logic1/4(Air_tAFS_mp)
  inlet air Minimum Logic1/1(AirHt_tRefair_mp) -> AirHt_tRefair_mp/1
  Air_tIntkVUs/1 -> inlet air Minimum Logic1/5(Air_tIntkVUs)
  CEngDsT_t/1 -> Minimum Logic/1(CEngDsT_t)
  DSM_bAirHtCEngDsT/1 -> Minimum Logic/4(DSM_bAirHtCEngDsT)
  DSM_bAirHtAFST/1 -> inlet air Minimum Logic1/8(DSM_bAirHtAFST)
  Minimum Logic/1(AirHt_tRef_mp) -> AirHt_tRef_mp/1
  FuelT_t/1 -> Minimum Logic/2(FuelT_t)
  Air_tCACDs_mp/1 -> inlet air Minimum Logic1/3(Air_tCACDs_mp)

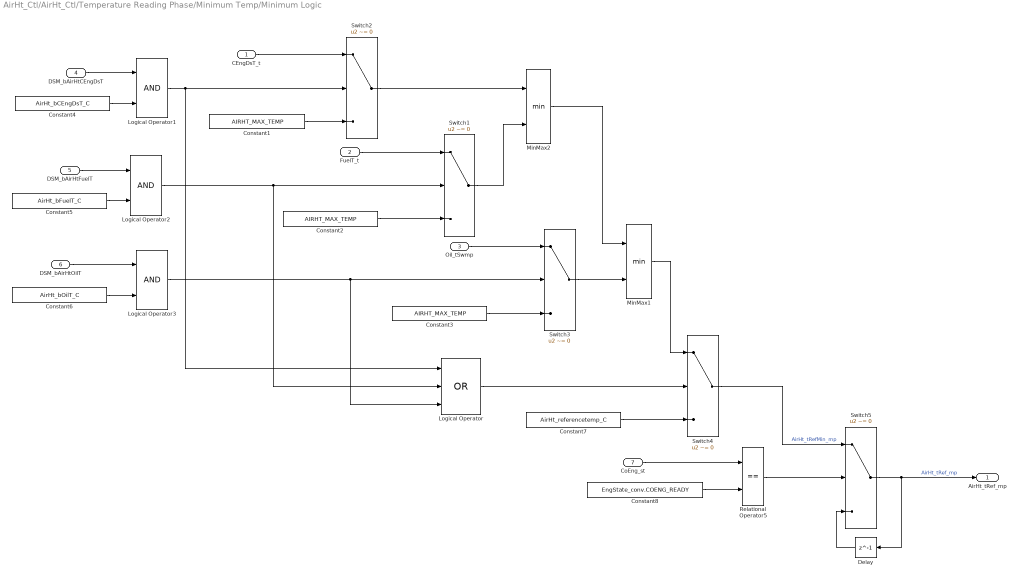
== system AirHt_Ctl/AirHt_Ctl/Temperature Reading Phase/Minimum Temp/Minimum Logic ==
  CEngDsT_t : Inport
  FuelT_t : Inport  Port=2
  Oil_tSwmp : Inport  Port=3
  DSM_bAirHtCEngDsT : Inport  Description=Status of FId_AirHtCEngDsT  Port=4
  DSM_bAirHtFuelT : Inport  Description=Status of FId_AirHtFuelT  Port=5
  DSM_bAirHtOilT : Inport  Description=Status of FId_AirHtOilT  Port=6
  CoEng_st : Inport  Port=7
  Constant1 : Constant  Value=AIRHT_MAX_TEMP  OutDataTypeStr=Inherit: Inherit via back propagation  SampleTime=-1
  Constant2 : Constant  Value=AIRHT_MAX_TEMP  OutDataTypeStr=Inherit: Inherit via back propagation  SampleTime=-1
  Constant3 : Constant  Value=AIRHT_MAX_TEMP  OutDataTypeStr=Inherit: Inherit via back propagation  SampleTime=-1
  Constant4 : Constant  Value=AirHt_bCEngDsT_C  SampleTime=-1
  Constant5 : Constant  Value=AirHt_bFuelT_C  SampleTime=-1
  Constant6 : Constant  Value=AirHt_bOilT_C  SampleTime=-1
  Constant7 : Constant  Value=AirHt_referencetemp_C  SampleTime=-1
  Constant8 : Constant  Value=EngState_conv.COENG_READY  SampleTime=-1
  Delay : Delay  DelayLength=1  InitialCondition=0
  Logical Operator : Logic  Operator=OR  Inputs=3  AllPortsSameDT=off  OutDataTypeStr=boolean
  Logical Operator1 : Logic  AllPortsSameDT=off  OutDataTypeStr=boolean
  Logical Operator2 : Logic  AllPortsSameDT=off  OutDataTypeStr=boolean
  Logical Operator3 : Logic  AllPortsSameDT=off  OutDataTypeStr=boolean
  MinMax1 : MinMax  Inputs=2  SaturateOnIntegerOverflow=on  InputSameDT=on
  MinMax2 : MinMax  Inputs=2  SaturateOnIntegerOverflow=on  InputSameDT=on
  Relational Operator5 : RelationalOperator  Operator===  OutDataTypeStr=boolean  RndMeth=Simplest  InputSameDT=on
  Switch1 : Switch  Criteria=u2 ~= 0  SaturateOnIntegerOverflow=on  InputSameDT=on
  Switch2 : Switch  Criteria=u2 ~= 0  InputSameDT=on
  Switch3 : Switch  Criteria=u2 ~= 0  SaturateOnIntegerOverflow=on  InputSameDT=on
  Switch4 : Switch  Criteria=u2 ~= 0  SaturateOnIntegerOverflow=on  InputSameDT=on
  Switch5 : Switch  Criteria=u2 ~= 0  InputSameDT=on
  AirHt_tRef_mp : Outport
  wires:
  Constant1/1 -> Switch2/3
  Logical Operator1/1 -> Logical Operator/1, Switch2/2
  Logical Operator3/1 -> Logical Operator/3, Switch3/2
  CEngDsT_t/1 -> Switch2/1
  Constant2/1 -> Switch1/3
  MinMax2/1 -> MinMax1/1
  Switch3/1 -> MinMax1/2
  Constant3/1 -> Switch3/3
  Oil_tSwmp/1 -> Switch3/1
  Switch1/1 -> MinMax2/2
  Switch2/1 -> MinMax2/1
  Logical Operator2/1 -> Logical Operator/2, Switch1/2
  FuelT_t/1 -> Switch1/1
  Switch4/1 -> Switch5/1  "AirHt_tRefMin_mp"
  MinMax1/1 -> Switch4/1
  Logical Operator/1 -> Switch4/2
  Constant7/1 -> Switch4/3
  DSM_bAirHtCEngDsT/1 -> Logical Operator1/1
  Constant4/1 -> Logical Operator1/2
  Constant5/1 -> Logical Operator2/2
  DSM_bAirHtFuelT/1 -> Logical Operator2/1
  DSM_bAirHtOilT/1 -> Logical Operator3/1
  Constant6/1 -> Logical Operator3/2
  Delay/1 -> Switch5/3
  Switch5/1 -> Delay/1, AirHt_tRef_mp/1  "AirHt_tRef_mp"
  Relational Operator5/1 -> Switch5/2
  CoEng_st/1 -> Relational Operator5/1
  Constant8/1 -> Relational Operator5/2

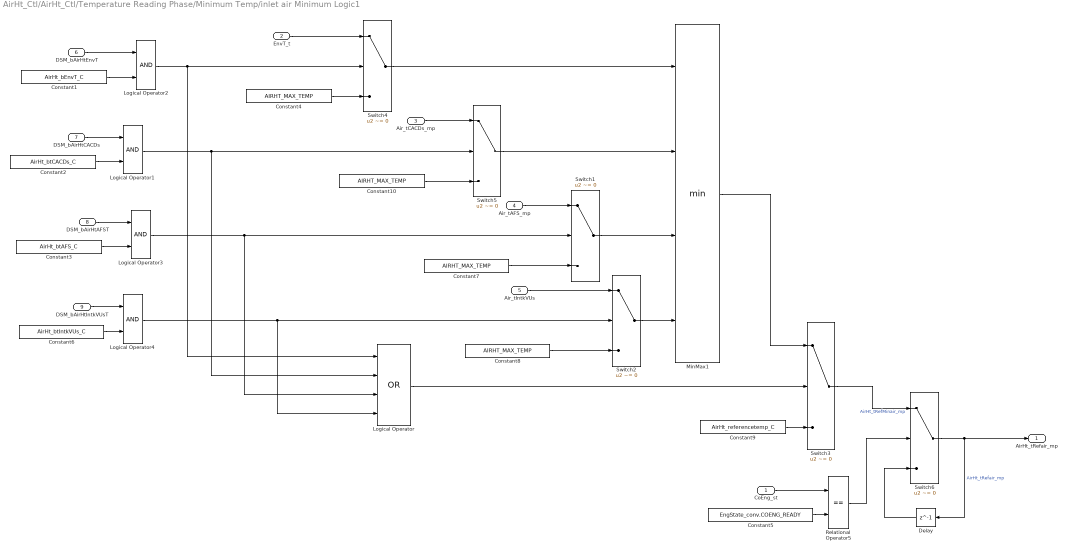
== system AirHt_Ctl/AirHt_Ctl/Temperature Reading Phase/Minimum Temp/inlet air Minimum Logic1 ==
  CoEng_st : Inport
  EnvT_t : Inport  Port=2
  Air_tCACDs_mp : Inport  Tag=deg  Description=Charge-air temperature downstream from charge-air cooler  Port=3
  Air_tAFS_mp : Inport  Tag=deg  Description=Induction air temperature at the HFM  Port=4
  Air_tIntkVUs : Inport  Tag=deg  Description=Intake air temperature upstream of the inlet valve  Port=5
  DSM_bAirHtEnvT : Inport  Description=Status of FId_AirHtEnvT_mp  Port=6
  DSM_bAirHtCACDs : Inport  Description=Status of FId_AirHtCACDs  Port=7
  DSM_bAirHtAFST : Inport  Description=Status of FId_AirHtEnvT_mp  Port=8
  DSM_bAirHtIntkVUsT : Inport  Description=Status of FId_AirHtCACDs  Port=9
  Constant1 : Constant  Value=AirHt_bEnvT_C  SampleTime=-1
  Constant{4,7..8,10} (4 alike) : Constant  Value=AIRHT_MAX_TEMP  OutDataTypeStr=Inherit: Inherit via back propagation  SampleTime=-1
  Constant2 : Constant  Value=AirHt_btCACDs_C  SampleTime=-1
  Constant3 : Constant  Value=AirHt_btAFS_C  SampleTime=-1
  Constant5 : Constant  Value=EngState_conv.COENG_READY  SampleTime=-1
  Constant6 : Constant  Value=AirHt_btIntkVUs_C  SampleTime=-1
  Constant9 : Constant  Value=AirHt_referencetemp_C  SampleTime=-1
  Delay : Delay  DelayLength=1  InitialCondition=0
  Logical Operator : Logic  Operator=OR  Inputs=4  AllPortsSameDT=off  OutDataTypeStr=boolean
  Logical Operator{1..4} (4 alike) : Logic  AllPortsSameDT=off  OutDataTypeStr=boolean
  MinMax1 : MinMax  Inputs=4  SaturateOnIntegerOverflow=on  InputSameDT=on
  Relational Operator5 : RelationalOperator  Operator===  OutDataTypeStr=boolean  RndMeth=Simplest  InputSameDT=on
  Switch{1..5} (5 alike) : Switch  Criteria=u2 ~= 0  SaturateOnIntegerOverflow=on  InputSameDT=on
  Switch6 : Switch  Criteria=u2 ~= 0  InputSameDT=on
  AirHt_tRefair_mp : Outport
  wires:
  Constant9/1 -> Switch3/3
  Switch3/1 -> Switch6/1  "AirHt_tRefMinair_mp"
  Delay/1 -> Switch6/3
  Switch6/1 -> AirHt_tRefair_mp/1, Delay/1  "AirHt_tRefair_mp"
  Relational Operator5/1 -> Switch6/2
  Logical Operator/1 -> Switch3/2
  MinMax1/1 -> Switch3/1
  CoEng_st/1 -> Relational Operator5/1
  Constant5/1 -> Relational Operator5/2
  DSM_bAirHtEnvT/1 -> Logical Operator2/1
  Constant2/1 -> Logical Operator1/2
  DSM_bAirHtAFST/1 -> Logical Operator3/1
  Constant7/1 -> Switch1/3
  Constant8/1 -> Switch2/3
  Logical Operator1/1 -> Logical Operator/2, Switch5/2
  Logical Operator2/1 -> Logical Operator/1, Switch4/2
  Constant10/1 -> Switch5/3
  Switch2/1 -> MinMax1/4
  Switch1/1 -> MinMax1/3
  Switch5/1 -> MinMax1/2
  Air_tAFS_mp/1 -> Switch1/1
  Constant4/1 -> Switch4/3
  Logical Operator3/1 -> Logical Operator/3, Switch1/2
  Logical Operator4/1 -> Logical Operator/4, Switch2/2
  Air_tIntkVUs/1 -> Switch2/1
  Switch4/1 -> MinMax1/1
  Air_tCACDs_mp/1 -> Switch5/1
  EnvT_t/1 -> Switch4/1
  Constant6/1 -> Logical Operator4/2
  DSM_bAirHtIntkVUsT/1 -> Logical Operator4/1
  DSM_bAirHtCACDs/1 -> Logical Operator1/1
  Constant1/1 -> Logical Operator2/2
  Constant3/1 -> Logical Operator3/2

== stateflow chart AirHt_Ctl/AirHt State Logic/AirHt State Calculation/Chart ==
  state HEAT
    state HEATING
      state STBHTR
        entry:
        AirHt_st =AirHtState_conv.AIRHT_STBHTR;
        AirHt_tiStByHtElapsed = AirHt_tiStByHtElapsed + DT;
        during:
        AirHt_tiStByHtElapsed = AirHt_tiStByHtElapsed + DT;
        exit:
        AirHt_stOld =AirHtState_conv.AIRHT_STBHTR;
      state PREHTR
        entry:
        AirHt_st =AirHtState_conv.AIRHT_PREHTR;
        AirHt_tiPreHtElapsed = AirHt_tiPreHtElapsed + DT;
        during:
        AirHt_tiPreHtElapsed = AirHt_tiPreHtElapsed + DT;
        exit:
        AirHt_stOld =AirHtState_conv.AIRHT_PREHTR;
      state CRKHTR
        entry:
        AirHt_st =AirHtState_conv.AIRHT_CRKHTR;
        AirHt_tiCrankHtElapsed = AirHt_tiCrankHtElapsed + DT;
        during:
        AirHt_tiCrankHtElapsed = AirHt_tiCrankHtElapsed + DT;
        exit:
        AirHt_stOld =AirHtState_conv.AIRHT_CRKHTR
      state STB
        entry:
        AirHt_st =AirHtState_conv.AIRHT_STB;
        exit:
        AirHt_stOld =AirHtState_conv.AIRHT_STB;
      state POSTHTR
        entry:
        AirHt_st =AirHtState_conv.AIRHT_POSTHTR;
        AirHt_tiPostHtElapsed = AirHt_tiPostHtElapsed + DT;
        during:
        AirHt_tiPostHtElapsed = AirHt_tiPostHtElapsed + DT;
        exit:
        AirHt_stOld =AirHtState_conv.AIRHT_END;
      state CRK
        entry:
        AirHt_st =AirHtState_conv.AIRHT_CRK;
        exit:
        AirHt_stOld =AirHtState_conv.AIRHT_CRK;
      (default) -> PREHTR
      PREHTR -> STBHTR [order 2] : [AirHt_tiPreHtElapsed >=AirHt_tiPreHt_mp]
          | {AirHt_tiPreHtElapsed=0;}
      STBHTR -> STB [order 2] : [AirHt_tiStByHtElapsed >=AirHt_tiStByHt_mp]
          | {AirHt_tiStByHtElapsed=0;}
      STBHTR -> CRKHTR [order 1] : [Epm_nEng> AirHt_nMin_C]
          | {AirHt_tiStByHtElapsed=0;}
      PREHTR -> CRKHTR [order 1] : [Epm_nEng> AirHt_nMin_C]
          | {AirHt_tiPreHtElapsed=0;}
      STB -> CRKHTR : [Epm_nEng> AirHt_nMin_C]
      CRKHTR -> POSTHTR [order 1] : [CoEng_st == EngState_conv.COENG_RUNNING]
          | {AirHt_tiCrankHtElapsed=0;}
      CRKHTR -> STB [order 2] : [Epm_nEng<= AirHt_nMin_C]
          | {AirHt_tiCrankHtElapsed=0;}
      CRK -> STB [order 2] : [Epm_nEng<= AirHt_nMin_C]
      CRKHTR -> CRK [order 3] : [AirHt_tiCrankHtElapsed >=AirHt_tiCrankHt_mp]
          | {AirHt_tiCrankHtElapsed=0;}
      CRK -> POSTHTR [order 1] : [CoEng_st ==EngState_conv.COENG_RUNNING]
    state END
      entry:
      AirHt_st =AirHtState_conv.AIRHT_END;
      exit:
      AirHt_stOld =AirHtState_conv.AIRHT_END;
    (default) -> HEATING
    POSTHTR -> END : [AirHt_tiPostHtElapsed >=AirHt_tiPostHt_mp]
        | {AirHt_tiPostHtElapsed=0;}
    HEATING -> END : [AirHt_stLowBatt_mp == 1]
  state READING
    entry:
    AirHt_st =AirHtState_conv.AIRHT_READING;
    during:
    AirHt_tiStDelay=AirHt_tiStDelay+DT;
    exit:
    AirHt_stOld =AirHtState_conv.AIRHT_READING;
  state AFTERRUN
    entry:
    AirHt_st =AirHtState_conv.AIRHT_AFTERRUN;
    exit:
    AirHt_stOld =AirHtState_conv.AIRHT_AFTERRUN;
  (default) -> READING
  READING -> HEAT [order 2] : [AirHt_tiStDelay>=AirHt_tiStDelay_C]
      | {Temp_Calc;AirHt_tiStDelay=0;}
  READING -> AFTERRUN [order 1] : [(CoEng_st ==EngState_conv.COENG_STOPPING) ||...
      | (CoEng_st ==EngState_conv.COENG_FINISH)]
  AFTERRUN -> READING : [(CoEng_st ==EngState_conv.COENG_READY) ||...
      | (CoEng_st ==EngState_conv.COENG_CRANKING)]
      | {AirHt_tiPostHtElapsed=0;
      | AirHt_tiCrankHtElapsed=0;
      | AirHt_tiStByHtElapsed=0;
      | AirHt_tiPreHtElapsed=0;}
  HEAT -> AFTERRUN : [(CoEng_st ==EngState_conv.COENG_STOPPING) ||...
      | (CoEng_st ==EngState_conv.COENG_FINISH)]
  data: T15_st input; CoEng_st input; AirHt_nMin_C input; AirHt_stLowBatt_mp input; Epm_nEng input; AirHt_tiPostHt_mp input; AirHt_tiCrankHt_mp input; AirHt_tiStByHt_mp input; AirHt_tiPreHt_mp input; AirHt_st output; AirHt_stOld output; DT input; AirHt_tiPreHtElapsed data_store_memory; AirHt_tiCrankHtElapsed data_store_memory; AirHt_tiPostHtElapsed data_store_memory; AirHt_tiStByHtElapsed data_store_memory; AirHt_tiStDelay data_store_memory; AirHt_tiStDelay_C input
  events: Temp_Calc output FUNCTION_CALL_EVENT
